simulink model "cell_balncing_with_code"  (R2019a)
settings: Solver=VariableStepAuto  StartTime=0.0  StopTime=2100  RelTol=1e-3
undefined symbols (not defined in the file): Ion, Lithium
libraries: powerlib x17, electricdrivelib x8
settings Model: Creator=chaser  LastModifiedBy=sujan
settings OptimizationCC: LifeSpan=inf
settings DebuggingCC: ArithmeticOperatorsInVariantConditions=warning
settings CodeAppCC: StateflowObjectComments=on

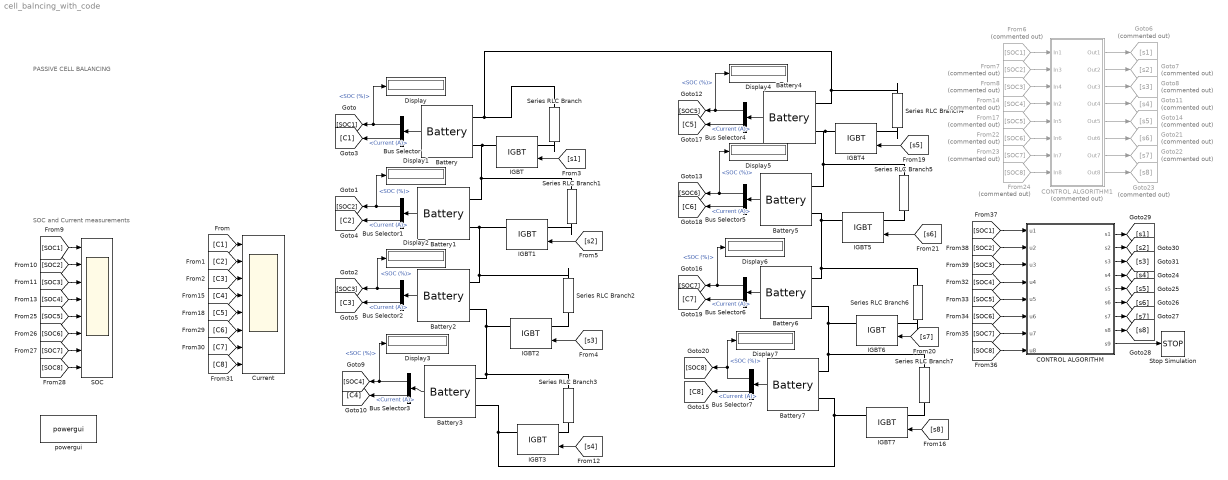
== system cell_balncing_with_code ==
  note: SOC and Current measurements
  note: PASSIVE CELL BALANCING
  Battery : electricdrivelib/Extra Sources/Battery  BatType=Lithium-Ion  ShowTempParam=off  ThermalPreset=no  ShowAgeParam=off  NomV=3.7  NomQ=2.6  SOC=80  Batt_Tr=10  PresetModel=on  MaxQ=2.6  MinV=2.775  FullV=4.3068  Dis_rate=1.1304  R=0.014231  Normal_OP=2.3513  expZone="[3.9974     0.12774]"  current=[6.5 13 32.5]  Units=Time  Tci=20  NomT=20  T2=-30  MaxQ2=4.8  FullV2=7.1  Normal_OP2=5.655  expZone2="[6.58           1]"  Rca=0.6  ti=2000  Dp=0  Neq0=0  Tsim=1e6  Ta1=25  Qeol=5.4*0.9  Reol=0.013333*1.2  Char_age=[2.3478, 3]  Dis_age=[2.3478, 10]  N1=1500  N2=10500  N3=1000  N4=1400  Ta2=45  N5=950
      settings: SourceProductName=Simscape Electrical
  Battery1 : electricdrivelib/Extra Sources/Battery  BatType=Lithium-Ion  ShowTempParam=off  ThermalPreset=no  ShowAgeParam=off  NomV=3.7  NomQ=2.6  SOC=70  Batt_Tr=10  PresetModel=on  MaxQ=2.6  MinV=2.775  FullV=4.3068  Dis_rate=1.1304  R=0.014231  Normal_OP=2.3513  expZone="[3.9974     0.12774]"  current=[6.5 13 32.5]  Units=Time  Tci=20  NomT=20  T2=-30  MaxQ2=4.8  FullV2=7.1  Normal_OP2=5.655  expZone2="[6.58           1]"  Rca=0.6  ti=2000  Dp=0  Neq0=0  Tsim=1e6  Ta1=25  Qeol=5.4*0.9  Reol=0.013333*1.2  Char_age=[2.3478, 3]  Dis_age=[2.3478, 10]  N1=1500  N2=10500  N3=1000  N4=1400  Ta2=45  N5=950
      settings: SourceProductName=Simscape Electrical
  Battery2 : electricdrivelib/Extra Sources/Battery  BatType=Lithium-Ion  ShowTempParam=off  ThermalPreset=no  ShowAgeParam=off  NomV=3.7  NomQ=2.6  SOC=60  Batt_Tr=10  PresetModel=on  MaxQ=2.6  MinV=2.775  FullV=4.3068  Dis_rate=1.1304  R=0.014231  Normal_OP=2.3513  expZone="[3.9974     0.12774]"  current=[6.5 13 32.5]  Units=Time  Tci=20  NomT=20  T2=-30  MaxQ2=4.8  FullV2=7.1  Normal_OP2=5.655  expZone2="[6.58           1]"  Rca=0.6  ti=2000  Dp=0  Neq0=0  Tsim=1e6  Ta1=25  Qeol=5.4*0.9  Reol=0.013333*1.2  Char_age=[2.3478, 3]  Dis_age=[2.3478, 10]  N1=1500  N2=10500  N3=1000  N4=1400  Ta2=45  N5=950
      settings: SourceProductName=Simscape Electrical
  Battery3 : electricdrivelib/Extra Sources/Battery  BatType=Lithium-Ion  ShowTempParam=off  ThermalPreset=no  ShowAgeParam=off  NomV=3.7  NomQ=2.6  SOC=20  Batt_Tr=10  PresetModel=on  MaxQ=2.6  MinV=2.775  FullV=4.3068  Dis_rate=1.1304  R=0.014231  Normal_OP=2.3513  expZone="[3.9974     0.12774]"  current=[6.5 13 32.5]  Units=Time  Tci=20  NomT=20  T2=-30  MaxQ2=4.8  FullV2=7.1  Normal_OP2=5.655  expZone2="[6.58           1]"  Rca=0.6  ti=2000  Dp=0  Neq0=0  Tsim=1e6  Ta1=25  Qeol=5.4*0.9  Reol=0.013333*1.2  Char_age=[2.3478, 3]  Dis_age=[2.3478, 10]  N1=1500  N2=10500  N3=1000  N4=1400  Ta2=45  N5=950
      settings: SourceProductName=Simscape Electrical
  Battery4 : electricdrivelib/Extra Sources/Battery  BatType=Lithium-Ion  ShowTempParam=off  ThermalPreset=no  ShowAgeParam=off  NomV=3.7  NomQ=2.6  SOC=80  Batt_Tr=10  PresetModel=on  MaxQ=2.6  MinV=2.775  FullV=4.3068  Dis_rate=1.1304  R=0.014231  Normal_OP=2.3513  expZone="[3.9974     0.12774]"  current=[6.5 13 32.5]  Units=Time  Tci=20  NomT=20  T2=-30  MaxQ2=4.8  FullV2=7.1  Normal_OP2=5.655  expZone2="[6.58           1]"  Rca=0.6  ti=2000  Dp=0  Neq0=0  Tsim=1e6  Ta1=25  Qeol=5.4*0.9  Reol=0.013333*1.2  Char_age=[2.3478, 3]  Dis_age=[2.3478, 10]  N1=1500  N2=10500  N3=1000  N4=1400  Ta2=45  N5=950
      settings: SourceProductName=Simscape Electrical
  Battery5 : electricdrivelib/Extra Sources/Battery  BatType=Lithium-Ion  ShowTempParam=off  ThermalPreset=no  ShowAgeParam=off  NomV=3.7  NomQ=2.6  SOC=70  Batt_Tr=10  PresetModel=on  MaxQ=2.6  MinV=2.775  FullV=4.3068  Dis_rate=1.1304  R=0.014231  Normal_OP=2.3513  expZone="[3.9974     0.12774]"  current=[6.5 13 32.5]  Units=Time  Tci=20  NomT=20  T2=-30  MaxQ2=4.8  FullV2=7.1  Normal_OP2=5.655  expZone2="[6.58           1]"  Rca=0.6  ti=2000  Dp=0  Neq0=0  Tsim=1e6  Ta1=25  Qeol=5.4*0.9  Reol=0.013333*1.2  Char_age=[2.3478, 3]  Dis_age=[2.3478, 10]  N1=1500  N2=10500  N3=1000  N4=1400  Ta2=45  N5=950
      settings: SourceProductName=Simscape Electrical
  Battery6 : electricdrivelib/Extra Sources/Battery  BatType=Lithium-Ion  ShowTempParam=off  ThermalPreset=no  ShowAgeParam=off  NomV=3.7  NomQ=2.6  SOC=60  Batt_Tr=10  PresetModel=on  MaxQ=2.6  MinV=2.775  FullV=4.3068  Dis_rate=1.1304  R=0.014231  Normal_OP=2.3513  expZone="[3.9974     0.12774]"  current=[6.5 13 32.5]  Units=Time  Tci=20  NomT=20  T2=-30  MaxQ2=4.8  FullV2=7.1  Normal_OP2=5.655  expZone2="[6.58           1]"  Rca=0.6  ti=2000  Dp=0  Neq0=0  Tsim=1e6  Ta1=25  Qeol=5.4*0.9  Reol=0.013333*1.2  Char_age=[2.3478, 3]  Dis_age=[2.3478, 10]  N1=1500  N2=10500  N3=1000  N4=1400  Ta2=45  N5=950
      settings: SourceProductName=Simscape Electrical
  Battery7 : electricdrivelib/Extra Sources/Battery  BatType=Lithium-Ion  ShowTempParam=off  ThermalPreset=no  ShowAgeParam=off  NomV=3.7  NomQ=2.6  SOC=20  Batt_Tr=10  PresetModel=on  MaxQ=2.6  MinV=2.775  FullV=4.3068  Dis_rate=1.1304  R=0.014231  Normal_OP=2.3513  expZone="[3.9974     0.12774]"  current=[6.5 13 32.5]  Units=Time  Tci=20  NomT=20  T2=-30  MaxQ2=4.8  FullV2=7.1  Normal_OP2=5.655  expZone2="[6.58           1]"  Rca=0.6  ti=2000  Dp=0  Neq0=0  Tsim=1e6  Ta1=25  Qeol=5.4*0.9  Reol=0.013333*1.2  Char_age=[2.3478, 3]  Dis_age=[2.3478, 10]  N1=1500  N2=10500  N3=1000  N4=1400  Ta2=45  N5=950
      settings: SourceProductName=Simscape Electrical
  Bus Selector{,1..7} (8 alike) : BusSelector  OutputSignals=SOC (%),Current (A)
  CONTROL ALGORITHM : MATLAB Function  TreatAsAtomicUnit=on
  CONTROL ALGORITHM1 : Subsystem  Commented=on
  Current : Scope  NumInputPorts=8
  Display{,1..7} (8 alike) : Display
  From14 : From  Commented=on  GotoTag=SOC4
  From17 : From  Commented=on  GotoTag=SOC5
  From22 : From  Commented=on  GotoTag=SOC6
  From23 : From  Commented=on  GotoTag=SOC7
  From24 : From  Commented=on  GotoTag=SOC8
  From6 : From  Commented=on  GotoTag=SOC1
  From7 : From  Commented=on  GotoTag=SOC2
  From8 : From  Commented=on  GotoTag=SOC3
  Goto11 : Goto  Commented=on  GotoTag=s4
  Goto14 : Goto  Commented=on  GotoTag=s5
  Goto21 : Goto  Commented=on  GotoTag=s6
  Goto22 : Goto  Commented=on  GotoTag=s7
  Goto23 : Goto  Commented=on  GotoTag=s8
  Goto6 : Goto  Commented=on  GotoTag=s1
  Goto7 : Goto  Commented=on  GotoTag=s2
  Goto8 : Goto  Commented=on  GotoTag=s3
  IGBT{,1..7} (8 alike) : powerlib/Power Electronics/IGBT  Ron=0.001  Lon=0  Vf=1  Tf=1e-6  Tt=2e-6  IC=0  Rs=1e-5  Cs=0  Measurements=on
      settings: SourceProductName=Simscape Electrical
  SOC : Scope  NumInputPorts=8
  Series RLC Branch{,1..7} (8 alike) : powerlib/Elements/Series RLC Branch  LConnTagsString=__new0  RConnTagsString=__new0  BranchType=R  Resistance=1  Inductance=1e-3  SetiL0=off  InitialCurrent=0  Capacitance=1e-6  Setx0=off  InitialVoltage=0  Measurements=None
      settings: SourceProductName=Simscape Electrical
  Stop Simulation : Stop
  powergui : powerlib/powergui  Priority=1  SimulationMode=Continuous  SampleTime=50e-6  frequency=60  Iterations=50  frequencyindice=0  Pbase=100e6  ErrMax=1e-4  UnitsV=kV  UnitsW=MW  buscounter=0  FunctionMessages=off  echomessages=off  EnableUseOfTLC=off  CurrentSourceSwitches=off  DisableSnubberDevices=off  DisableRonSwitches=off  DisableVfSwitches=off  DisplayEquations=off  AutomaticDiscreteSolvers=off  SolverType=Tustin/Backward Euler (TBE)  Interpol=off  ExternalGateDelay=off  methode=off  Ts=100  x0status=blocks  SPID=on  SwTol=0  HookPort=off  NonlinearTolerance=1e-4  nMaxIteration=100  ContinueOnMaxIteration=off  RestoreLinks=warning  ResistiveCurrentMeasurement=off  Frange=[0:2:500]  Ylog=off  Xlog=on  ShowGrid=off  save=off  variable=ZData  structure=0  ZoomFFT=off  StartTime=0.0  cycles=1  DisplayStyle=1  fundamental=60  FreqAxis=off  MaxFrequency=1000  frequencyindicesteady=1  RmsSteady=1  display=off
      settings: SourceProductName=Simscape Electrical
  wires:
  [SOC5] -> SOC/5
  Bus Selector1/1 -> Display1/1, [SOC2]  "<SOC (%)>"
  [s4] -> IGBT3/1
  Battery6/1 -> Bus Selector6/1
  [SOC6] -> SOC/6
  [SOC3] -> SOC/3
  [C6] -> Current/6
  Bus Selector5/1 -> Display5/1, [SOC6]  "<SOC (%)>"
  Battery3/1 -> Bus Selector3/1
  Bus Selector/2 -> [C1]  "<Current (A)>"
  [SOC4] -> SOC/4
  [SOC1] -> SOC/1
  Bus Selector6/1 -> Display6/1, [SOC7]  "<SOC (%)>"
  [C7] -> Current/7
  [s1] -> IGBT/1
  Bus Selector3/2 -> [C4]  "<Current (A)>"
  [s8] -> IGBT7/1
  [s2] -> IGBT1/1
  [SOC8] -> SOC/8
  Bus Selector7/1 -> Display7/1, [SOC8]  "<SOC (%)>"
  [C8] -> Current/8
  [s6] -> IGBT5/1
  Battery4/1 -> Bus Selector4/1
  Bus Selector7/2 -> [C8]  "<Current (A)>"
  Bus Selector6/2 -> [C7]  "<Current (A)>"
  Bus Selector5/2 -> [C6]  "<Current (A)>"
  Battery5/1 -> Bus Selector5/1
  Bus Selector4/2 -> [C5]  "<Current (A)>"
  [C2] -> Current/2
  Bus Selector4/1 -> Display4/1, [SOC5]  "<SOC (%)>"
  [s5] -> IGBT4/1
  Battery7/1 -> Bus Selector7/1
  Battery/1 -> Bus Selector/1
  Battery1/1 -> Bus Selector1/1
  [s3] -> IGBT2/1
  Battery2/1 -> Bus Selector2/1
  Bus Selector2/1 -> Display2/1, [SOC3]  "<SOC (%)>"
  [SOC2] -> SOC/2
  Bus Selector/1 -> Display/1, [SOC1]  "<SOC (%)>"
  Bus Selector3/1 -> Display3/1, [SOC4]  "<SOC (%)>"
  Bus Selector1/2 -> [C2]  "<Current (A)>"
  Bus Selector2/2 -> [C3]  "<Current (A)>"
  [C3] -> Current/3
  [C4] -> Current/4
  [C5] -> Current/5
  [s7] -> IGBT6/1
  [SOC7] -> SOC/7
  [C1] -> Current/1
  [SOC2] -> CONTROL ALGORITHM/2(u2)
  [SOC3] -> CONTROL ALGORITHM/3(u3)
  [SOC5] -> CONTROL ALGORITHM/5(u5)
  [SOC6] -> CONTROL ALGORITHM/6(u6)
  [SOC4] -> CONTROL ALGORITHM/4(u4)
  [SOC1] -> CONTROL ALGORITHM/1(u1)
  [SOC7] -> CONTROL ALGORITHM/7(u7)
  [SOC8] -> CONTROL ALGORITHM/8(u8)
  CONTROL ALGORITHM/3(s3) -> [s3]
  CONTROL ALGORITHM/6(s6) -> [s6]
  CONTROL ALGORITHM/5(s5) -> [s5]
  CONTROL ALGORITHM/2(s2) -> [s2]
  CONTROL ALGORITHM/8(s8) -> [s8]
  CONTROL ALGORITHM/7(s7) -> [s7]
  CONTROL ALGORITHM/1(s1) -> [s1]
  CONTROL ALGORITHM/4(s4) -> [s4]
  CONTROL ALGORITHM/9(s9) -> Stop Simulation/1
  CONTROL ALGORITHM1/8(Out8) -> Goto23/1
  From24/1 -> CONTROL ALGORITHM1/8(In8)
  CONTROL ALGORITHM1/5(Out5) -> Goto14/1
  CONTROL ALGORITHM1/7(Out7) -> Goto22/1
  From7/1 -> CONTROL ALGORITHM1/2(In3)
  CONTROL ALGORITHM1/1(Out1) -> Goto6/1
  CONTROL ALGORITHM1/4(Out4) -> Goto11/1
  From17/1 -> CONTROL ALGORITHM1/5(In5)
  From22/1 -> CONTROL ALGORITHM1/6(In6)
  CONTROL ALGORITHM1/2(Out2) -> Goto7/1
  From23/1 -> CONTROL ALGORITHM1/7(In7)
  CONTROL ALGORITHM1/6(Out6) -> Goto21/1
  CONTROL ALGORITHM1/3(Out3) -> Goto8/1
  From6/1 -> CONTROL ALGORITHM1/1(In1)
  From8/1 -> CONTROL ALGORITHM1/3(In4)
  From14/1 -> CONTROL ALGORITHM1/4(In2)
  connections:
  IGBT7/RConn1 -- Battery7/LConn2 -- Battery3/LConn2 -- IGBT3/RConn1
  Series RLC Branch7/LConn1 -- IGBT6/RConn1 -- Battery6/LConn2 -- Battery7/LConn1
  Series RLC Branch6/LConn1 -- Battery6/LConn1 -- Battery5/LConn2 -- IGBT5/RConn1
  Battery/LConn2 -- Battery1/LConn1 -- Series RLC Branch1/LConn1 -- IGBT/RConn1
  Series RLC Branch/LConn1 -- Battery/LConn1 -- Series RLC Branch4/LConn1 -- Battery4/LConn1
  IGBT2/RConn1 -- Series RLC Branch3/LConn1 -- Battery3/LConn1 -- Battery2/LConn2
  Battery4/LConn2 -- Battery5/LConn1 -- Series RLC Branch5/LConn1 -- IGBT4/RConn1
  Series RLC Branch2/LConn1 -- Battery2/LConn1 -- Battery1/LConn2 -- IGBT1/RConn1
  Series RLC Branch1/RConn1 -- IGBT1/LConn1
  Series RLC Branch6/RConn1 -- IGBT6/LConn1
  Series RLC Branch7/RConn1 -- IGBT7/LConn1
  Series RLC Branch5/RConn1 -- IGBT5/LConn1
  Series RLC Branch3/RConn1 -- IGBT3/LConn1
  Series RLC Branch2/RConn1 -- IGBT2/LConn1
  Series RLC Branch/RConn1 -- IGBT/LConn1
  Series RLC Branch4/RConn1 -- IGBT4/LConn1

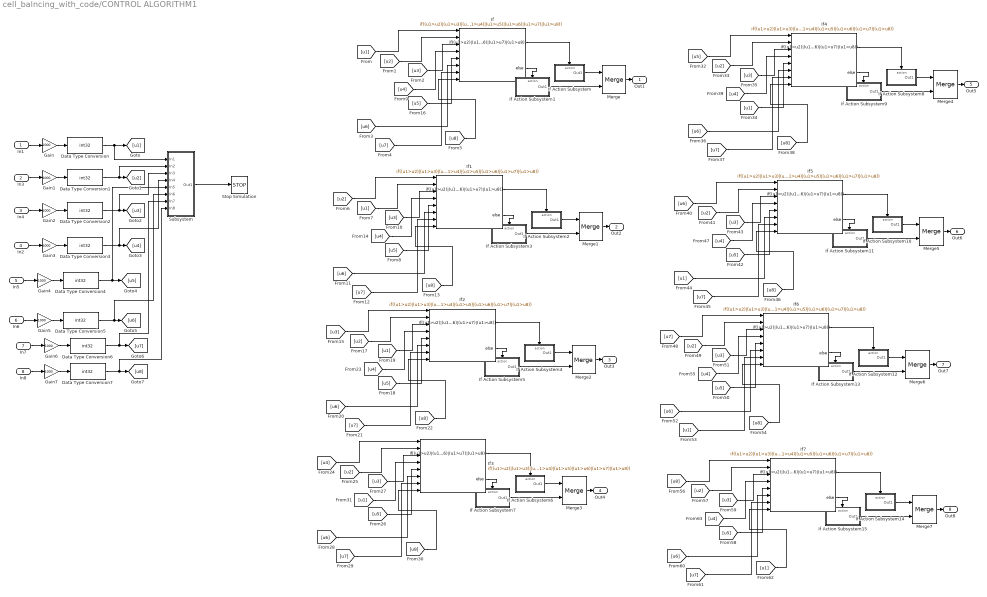
== system cell_balncing_with_code/CONTROL ALGORITHM1 ==
  In1 : Inport
  In3 : Inport  Port=2
  In4 : Inport  Port=3
  In2 : Inport  Port=4
  In5 : Inport  Port=5
  In6 : Inport  Port=6
  In7 : Inport  Port=7
  In8 : Inport  Port=8
  Data Type Conversion{,1..7} (8 alike) : DataTypeConversion  OutDataTypeStr=int32
  Gain{,1..7} (8 alike) : Gain  Gain=1000
  If{,1..7} (8 alike) : If  NumInputs=8  IfExpression=(u1>u2)|(u1>u3)|(u1>u4)|(u1>u5)|(u1>u6)|(u1>u7)|(u1>u8)
  If Action Subsystem : Subsystem  TreatAsAtomicUnit=on
  If Action Subsystem1 : Subsystem  TreatAsAtomicUnit=on
  If Action Subsystem10 : Subsystem  TreatAsAtomicUnit=on
  If Action Subsystem11 : Subsystem  TreatAsAtomicUnit=on
  If Action Subsystem12 : Subsystem  TreatAsAtomicUnit=on
  If Action Subsystem13 : Subsystem  TreatAsAtomicUnit=on
  If Action Subsystem14 : Subsystem  TreatAsAtomicUnit=on
  If Action Subsystem15 : Subsystem  TreatAsAtomicUnit=on
  If Action Subsystem2 : Subsystem  TreatAsAtomicUnit=on
  If Action Subsystem3 : Subsystem  TreatAsAtomicUnit=on
  If Action Subsystem4 : Subsystem  TreatAsAtomicUnit=on
  If Action Subsystem5 : Subsystem  TreatAsAtomicUnit=on
  If Action Subsystem6 : Subsystem  TreatAsAtomicUnit=on
  If Action Subsystem7 : Subsystem  TreatAsAtomicUnit=on
  If Action Subsystem8 : Subsystem  TreatAsAtomicUnit=on
  If Action Subsystem9 : Subsystem  TreatAsAtomicUnit=on
  Merge{,1..7} (8 alike) : Merge
  Stop Simulation : Stop
  Subsystem : Subsystem
  Out1 : Outport
  Out2 : Outport  Port=2
  Out3 : Outport  Port=3
  Out4 : Outport  Port=4
  Out5 : Outport  Port=5
  Out6 : Outport  Port=6
  Out7 : Outport  Port=7
  Out8 : Outport  Port=8
  wires:
  Gain/1 -> Data Type Conversion/1
  If Action Subsystem/1(Out1) -> Merge/1
  [u2] -> If/2
  If Action Subsystem1/1(Out1) -> Merge/2
  In1/1 -> Gain/1
  [u3] -> If/3
  If/1 -> If Action Subsystem/Action
  In3/1 -> Gain1/1
  Data Type Conversion2/1 -> Subsystem/3(In3), [u3]
  Data Type Conversion1/1 -> Subsystem/2(In2), [u2]
  Merge/1 -> Out1/1
  In4/1 -> Gain2/1
  Gain1/1 -> Data Type Conversion1/1
  Data Type Conversion/1 -> Subsystem/1(In1), [u1]
  If/2 -> If Action Subsystem1/Action
  Gain2/1 -> Data Type Conversion2/1
  Subsystem/1(Out1) -> Stop Simulation/1
  [u1] -> If/1
  Data Type Conversion3/1 -> Subsystem/4(In4), [u4]
  Gain3/1 -> Data Type Conversion3/1
  In2/1 -> Gain3/1
  [u4] -> If/4
  In5/1 -> Gain4/1
  Data Type Conversion4/1 -> Subsystem/5(In5), [u5]
  Gain4/1 -> Data Type Conversion4/1
  [u5] -> If/5
  Gain5/1 -> Data Type Conversion5/1
  Data Type Conversion5/1 -> Subsystem/6(In6), [u6]
  In6/1 -> Gain5/1
  Gain6/1 -> Data Type Conversion6/1
  Data Type Conversion6/1 -> Subsystem/7(In7), [u7]
  In7/1 -> Gain6/1
  Gain7/1 -> Data Type Conversion7/1
  Data Type Conversion7/1 -> Subsystem/8(In8), [u8]
  In8/1 -> Gain7/1
  [u6] -> If/6
  [u7] -> If/7
  [u8] -> If/8
  [u7] -> If1/7
  [u5] -> If1/5
  [u8] -> If1/8
  If1/1 -> If Action Subsystem2/Action
  [u3] -> If1/3
  If1/2 -> If Action Subsystem3/Action
  [u2] -> If1/1
  If Action Subsystem3/1(Out1) -> Merge1/2
  Merge1/1 -> Out2/1
  [u6] -> If1/6
  If Action Subsystem2/1(Out1) -> Merge1/1
  [u4] -> If1/4
  [u1] -> If1/2
  [u7] -> If2/7
  [u5] -> If2/5
  [u8] -> If2/8
  If2/1 -> If Action Subsystem4/Action
  [u1] -> If2/3
  If2/2 -> If Action Subsystem5/Action
  [u3] -> If2/1
  If Action Subsystem5/1(Out1) -> Merge2/2
  Merge2/1 -> Out3/1
  [u6] -> If2/6
  If Action Subsystem4/1(Out1) -> Merge2/1
  [u4] -> If2/4
  [u2] -> If2/2
  [u7] -> If3/7
  [u5] -> If3/5
  [u8] -> If3/8
  If3/1 -> If Action Subsystem6/Action
  [u3] -> If3/3
  If3/2 -> If Action Subsystem7/Action
  [u4] -> If3/1
  If Action Subsystem7/1(Out1) -> Merge3/2
  Merge3/1 -> Out4/1
  [u6] -> If3/6
  If Action Subsystem6/1(Out1) -> Merge3/1
  [u1] -> If3/4
  [u2] -> If3/2
  [u7] -> If4/7
  [u1] -> If4/5
  [u8] -> If4/8
  If4/1 -> If Action Subsystem8/Action
  [u3] -> If4/3
  If4/2 -> If Action Subsystem9/Action
  [u5] -> If4/1
  If Action Subsystem9/1(Out1) -> Merge4/2
  Merge4/1 -> Out5/1
  [u6] -> If4/6
  If Action Subsystem8/1(Out1) -> Merge4/1
  [u4] -> If4/4
  [u2] -> If4/2
  [u7] -> If5/7
  [u5] -> If5/5
  [u8] -> If5/8
  If5/1 -> If Action Subsystem10/Action
  [u3] -> If5/3
  If5/2 -> If Action Subsystem11/Action
  [u6] -> If5/1
  If Action Subsystem11/1(Out1) -> Merge5/2
  Merge5/1 -> Out6/1
  [u1] -> If5/6
  If Action Subsystem10/1(Out1) -> Merge5/1
  [u4] -> If5/4
  [u2] -> If5/2
  [u1] -> If6/7
  [u5] -> If6/5
  [u8] -> If6/8
  If6/1 -> If Action Subsystem12/Action
  [u3] -> If6/3
  If6/2 -> If Action Subsystem13/Action
  [u7] -> If6/1
  If Action Subsystem13/1(Out1) -> Merge6/2
  Merge6/1 -> Out7/1
  [u6] -> If6/6
  If Action Subsystem12/1(Out1) -> Merge6/1
  [u4] -> If6/4
  [u2] -> If6/2
  [u7] -> If7/7
  [u5] -> If7/5
  [u1] -> If7/8
  If7/1 -> If Action Subsystem14/Action
  [u3] -> If7/3
  If7/2 -> If Action Subsystem15/Action
  [u8] -> If7/1
  If Action Subsystem15/1(Out1) -> Merge7/2
  Merge7/1 -> Out8/1
  [u6] -> If7/6
  If Action Subsystem14/1(Out1) -> Merge7/1
  [u4] -> If7/4
  [u2] -> If7/2

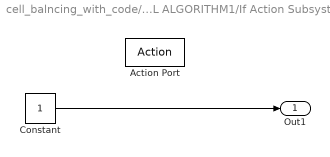
== system cell_balncing_with_code/CONTROL ALGORITHM1/If Action Subsystem ==
  Action Port : ActionPort
  Constant : Constant
  Out1 : Outport
  wires:
  Constant/1 -> Out1/1

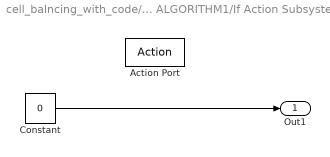
== system cell_balncing_with_code/CONTROL ALGORITHM1/If Action Subsystem1 ==
  Action Port : ActionPort
  Constant : Constant  Value=0
  Out1 : Outport
  wires:
  Constant/1 -> Out1/1

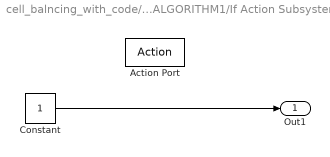
== system cell_balncing_with_code/CONTROL ALGORITHM1/If Action Subsystem10 ==
  Action Port : ActionPort
  Constant : Constant
  Out1 : Outport
  wires:
  Constant/1 -> Out1/1

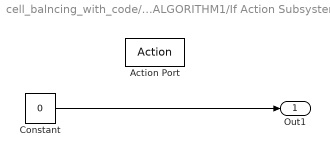
== system cell_balncing_with_code/CONTROL ALGORITHM1/If Action Subsystem11 ==
  Action Port : ActionPort
  Constant : Constant  Value=0
  Out1 : Outport
  wires:
  Constant/1 -> Out1/1

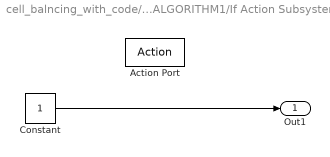
== system cell_balncing_with_code/CONTROL ALGORITHM1/If Action Subsystem12 ==
  Action Port : ActionPort
  Constant : Constant
  Out1 : Outport
  wires:
  Constant/1 -> Out1/1

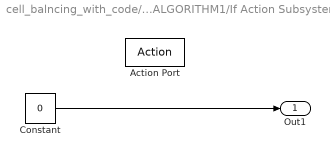
== system cell_balncing_with_code/CONTROL ALGORITHM1/If Action Subsystem13 ==
  Action Port : ActionPort
  Constant : Constant  Value=0
  Out1 : Outport
  wires:
  Constant/1 -> Out1/1

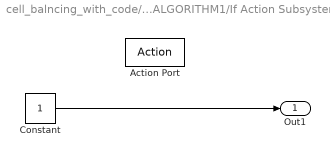
== system cell_balncing_with_code/CONTROL ALGORITHM1/If Action Subsystem14 ==
  Action Port : ActionPort
  Constant : Constant
  Out1 : Outport
  wires:
  Constant/1 -> Out1/1

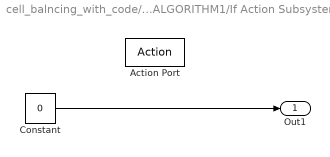
== system cell_balncing_with_code/CONTROL ALGORITHM1/If Action Subsystem15 ==
  Action Port : ActionPort
  Constant : Constant  Value=0
  Out1 : Outport
  wires:
  Constant/1 -> Out1/1

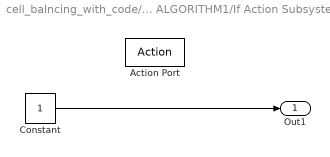
== system cell_balncing_with_code/CONTROL ALGORITHM1/If Action Subsystem2 ==
  Action Port : ActionPort
  Constant : Constant
  Out1 : Outport
  wires:
  Constant/1 -> Out1/1

== system cell_balncing_with_code/CONTROL ALGORITHM1/If Action Subsystem3 ==
  Action Port : ActionPort
  Constant : Constant  Value=0
  Out1 : Outport
  wires:
  Constant/1 -> Out1/1

== system cell_balncing_with_code/CONTROL ALGORITHM1/If Action Subsystem4 ==
  Action Port : ActionPort
  Constant : Constant
  Out1 : Outport
  wires:
  Constant/1 -> Out1/1

== system cell_balncing_with_code/CONTROL ALGORITHM1/If Action Subsystem5 ==
  Action Port : ActionPort
  Constant : Constant  Value=0
  Out1 : Outport
  wires:
  Constant/1 -> Out1/1

== system cell_balncing_with_code/CONTROL ALGORITHM1/If Action Subsystem6 ==
  Action Port : ActionPort
  Constant : Constant
  Out1 : Outport
  wires:
  Constant/1 -> Out1/1

== system cell_balncing_with_code/CONTROL ALGORITHM1/If Action Subsystem7 ==
  Action Port : ActionPort
  Constant : Constant  Value=0
  Out1 : Outport
  wires:
  Constant/1 -> Out1/1

== system cell_balncing_with_code/CONTROL ALGORITHM1/If Action Subsystem8 ==
  Action Port : ActionPort
  Constant : Constant
  Out1 : Outport
  wires:
  Constant/1 -> Out1/1

== system cell_balncing_with_code/CONTROL ALGORITHM1/If Action Subsystem9 ==
  Action Port : ActionPort
  Constant : Constant  Value=0
  Out1 : Outport
  wires:
  Constant/1 -> Out1/1

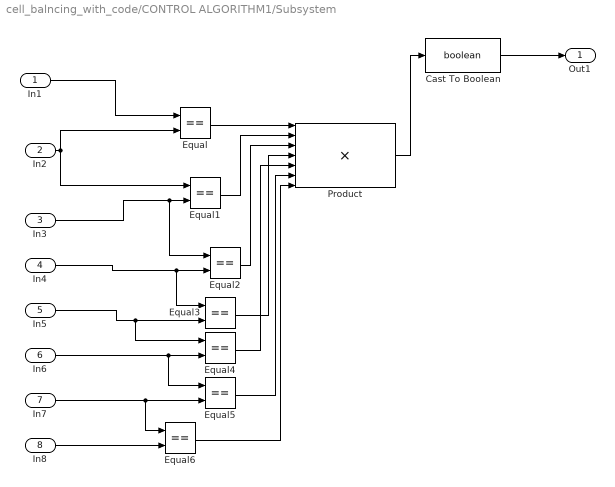
== system cell_balncing_with_code/CONTROL ALGORITHM1/Subsystem ==
  In1 : Inport
  In2 : Inport  Port=2
  In3 : Inport  Port=3
  In4 : Inport  Port=4
  In5 : Inport  Port=5
  In6 : Inport  Port=6
  In7 : Inport  Port=7
  In8 : Inport  Port=8
  Cast To Boolean : DataTypeConversion  OutDataTypeStr=boolean
  Equal{,1..6} (7 alike) : RelationalOperator  Operator===  OutDataTypeStr=boolean  RndMeth=Nearest
  Product : Product  Inputs=7
  Out1 : Outport
  wires:
  Equal1/1 -> Product/2
  Product/1 -> Cast To Boolean/1
  Equal/1 -> Product/1
  In3/1 -> Equal2/1, Equal1/2
  In2/1 -> Equal1/1, Equal/2
  In1/1 -> Equal/1
  Cast To Boolean/1 -> Out1/1
  In4/1 -> Equal3/1, Equal2/2
  Equal2/1 -> Product/3
  In5/1 -> Equal4/1, Equal3/2
  Equal3/1 -> Product/4
  In6/1 -> Equal5/1, Equal4/2
  Equal4/1 -> Product/5
  In7/1 -> Equal6/1, Equal5/2
  Equal5/1 -> Product/6
  In8/1 -> Equal6/2
  Equal6/1 -> Product/7

== matlab function cell_balncing_with_code/CONTROL ALGORITHM ==
  data: u1 input; s1 output; u2 input; u3 input; s2 output; s3 output; s4 output; u4 input; u5 input; u6 input; u7 input; u8 input; s5 output; s6 output; s7 output; s8 output; s9 output
function [s1,s2,s3,s4,s5,s6,s7,s8,s9] = fcn(u1,u2,u3,u4,u5,u6,u7,u8)


u1=u1*1000;
u2=u2*1000;
u3=u3*1000;
u4=u4*1000;
u5=u5*1000;
u6=u6*1000;
u7=u7*1000;
u8=u8*1000;


u1=int32(u1);
u2=int32(u2);
u3=int32(u3);
u4=int32(u4);
u5=int32(u5);
u6=int32(u6);
u7=int32(u7);
u8=int32(u8);


if((u1>u2)||(u1>u3)||(u1>u4)||(u1>u5)||(u1>u6)||(u1>u7)||(u1>u8))
    s1=1;
else
    s1=0;
end    

if((u2>u1)||(u2>u3)||(u2>u4)||(u2>u5)||(u2>u6)||(u2>u7)||(u2>u8))
    s2=1;
else
    s2=0;
end  

if((u3>u2)||(u3>u1)||(u3>u4)||(u3>u5)||(u3>u6)||(u3>u7)||(u3>u8))
    s3=1;
else
    s3=0;
end  

if((u4>u2)||(u4>u3)||(u4>u1)||(u4>u5)||(u4>u6)||(u4>u7)||(u4>u8))
    s4=1;
else
    s4=0;
end  

if((u5>u2)||(u5>u3)||(u5>u4)||(u5>u1)||(u5>u6)||(u5>u7)||(u5>u8))
    s5=1;
else
    s5=0;
end  

if((u6>u2)||(u6>u3)||(u6>u4)||(u6>u5)||(u6>u1)||(u6>u7)||(u6>u8))
    s6=1;
else
    s6=0;
end  

if((u7>u2)||(u7>u3)||(u7>u4)||(u7>u5)||(u7>u6)||(u7>u7)||(u7>u8))
    s7=1;
else
    s7=0;
end  

if((u8>u2)||(u8>u3)||(u8>u4)||(u8>u5)||(u8>u6)||(u8>u7)||(u8>u1))
    s8=1;
else
    s8=0;
end  

if((u1==u2)&&(u2==u3)&&(u3==u4)&&(u4==u5)&&(u5==u6)&&(u6==u7)&&(u7==u8))
    s9=1;
else
    s9=0;

end
